simulink model "MassSpringDamperTransferFuntion"  (R2020a)
settings: Solver=VariableStepAuto  StartTime=0.0  StopTime=10.0  MaxStep=0.01  RelTol=1e-3
values from neighbouring files (symbols this model uses):
  b = 1    [systemparameter.m]
  F = 10    [systemparameter.m]
  k = 20    [systemparameter.m]
  M = 1    [systemparameter.m]
libraries: dspsrcs4 x1
settings Model: Creator=diogo  LastModifiedBy=diogo

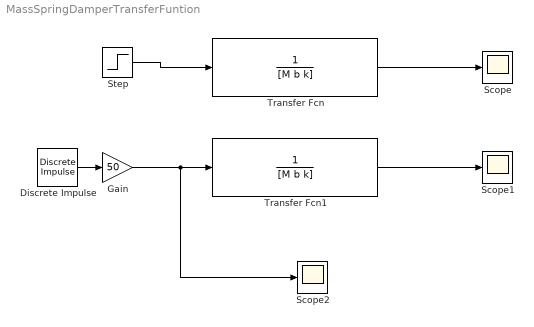
== system MassSpringDamperTransferFuntion ==
  Discrete Impulse : dspsrcs4/Discrete  Impulse  Delay=0  SampleTime=1  FrameSample=1  OutputFrames=off  dataType=double  isSigned=on  wordLen=16  udDataType=sfix(16)  fracBitsMode=Best precision  numFracBits=15  OutDataTypeStr=double  LastOutDataTypeStr=double
  Gain : Gain  Gain=50
  Scope : Scope
  Scope1 : Scope
  Scope2 : Scope
  Step : Step  After=F  SampleTime=0
  Transfer Fcn : TransferFcn  Denominator=[M b k]
  Transfer Fcn1 : TransferFcn  Denominator=[M b k]
  wires:
  Step/1 -> Transfer Fcn/1
  Transfer Fcn/1 -> Scope/1
  Transfer Fcn1/1 -> Scope1/1
  Discrete Impulse/1 -> Gain/1
  Gain/1 -> Scope2/1, Transfer Fcn1/1
